simulink model "V1MatlabWs"  (R2019b)
settings: Solver=FixedStepAuto  StartTime=0.0  StopTime=20.0  FixedStep=0.1  MaxStep=0.1  MinStep=0.1  RelTol=1e-3  EnableMultiTasking=on
values from neighbouring files (symbols this model uses):
  c1 = c    (= 1)    [V1SetParam.m]    (also in V3VektorSetParam.m; V7Callback_2018_05_25_18_20_53_343.mat; V7SetParam.m; myData.mat)
  c2 = c    (= 1)    [V1SetParam.m]    (also in V3VektorSetParam.m; V7Callback_2018_05_25_18_20_53_343.mat; V7SetParam.m)
  c3 = c    (= 1)    [V1SetParam.m]    (also in V3VektorSetParam.m; V7Callback_2018_05_25_18_20_53_343.mat; V7SetParam.m)
  c4 = c    (= 1)    [V1SetParam.m]    (also in V3VektorSetParam.m; V7Callback_2018_05_25_18_20_53_343.mat; V7SetParam.m)
  m1 = m    (= 2)    [V1SetParam.m]    (also in V3VektorSetParam.m; V7Callback_2018_05_25_18_20_53_343.mat; V7SetParam.m; myData.mat)
  m2 = m    (= 2)    [V1SetParam.m]    (also in V3VektorSetParam.m; V7Callback_2018_05_25_18_20_53_343.mat; V7SetParam.m)
  m3 = m    (= 2)    [V1SetParam.m]    (also in V3VektorSetParam.m; V7Callback_2018_05_25_18_20_53_343.mat; V7SetParam.m)
  v1 = 0    [V7Callback_2018_05_25_18_20_53_343.mat]    (also in V7SetParam.m)
  v2 = 0    [V7Callback_2018_05_25_18_20_53_343.mat]    (also in V7SetParam.m)
  v3 = 0    [V7Callback_2018_05_25_18_20_53_343.mat]    (also in V7SetParam.m)
  x1 = -1    [V7Callback_2018_05_25_18_20_53_343.mat]    (also in V7SetParam.m)
  x2 = 0    [V7Callback_2018_05_25_18_20_53_343.mat]    (also in V7SetParam.m)
  x3 = 1    [V7Callback_2018_05_25_18_20_53_343.mat]    (also in V7SetParam.m)
settings Model: Creator=Reichl  LastModifiedBy=jakob
settings DataIOCC: SaveFormat=Array  SignalLoggingSaveFormat=ModelDataLogs  ReturnWorkspaceOutputs=off
settings OptimizationCC: ExpressionDepthLimit=2147483647  LifeSpan=inf
settings DebuggingCC: UnderspecifiedInitializationDetection=Classic  MergeDetectMultiDrivingBlocksExec=none  SolverPrmCheckMsg=warning  FcnCallInpInsideContextMsg=warning  AllowSymbolicDim=off  StateNameClashWarn=warning  SFUnexpectedBacktrackingDiag=warning  SFNoUnconditionalDefaultTransitionDiag=warning  SFExecutionAtInitializationDiag=none  ArithmeticOperatorsInVariantConditions=warning
settings HardwareCC: ProdBitPerPointer=32  ProdBitPerSizeT=32  ProdBitPerPtrDiffT=32  ProdLargestAtomicFloat=None  ProdIntDivRoundTo=Undefined  ProdEndianess=Unspecified  ProdWordSize=32  ProdHWDeviceType=32-bit Generic
settings ModelReferenceCC: PropagateSignalLabelsOutOfModel=off
settings SFSimCC: SimUseLocalCustomCode=off  CustomCodeUndefinedFunction=UseInterfaceOnly
settings RTWCC: RTWUseLocalCustomCode=off
settings CodeAppCC: StateflowObjectComments=on
settings GRTTargetCC: TargetLangStandard=C89/C90 (ANSI)  GeneratePreprocessorConditionals=Disable all  CombineOutputUpdateFcns=off  GRTInterface=on
settings ConfigComp: CovMetricSettings=dw  CovHtmlReporting=on  CovSaveCumulativeToWorkspaceVar=on  CovSaveSingleToWorkspaceVar=on  CovExternalEMLEnable=off  CovSFcnEnable=off

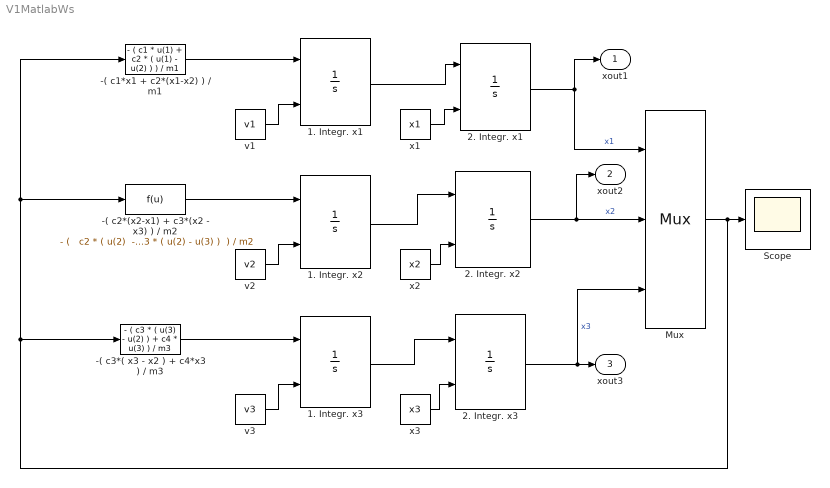
== system V1MatlabWs ==
  -( c1*x1 + c2*(x1-x2) ) / m1 : Fcn  Expr="- (   c1 * u(1)  +  c2 * ( u(1) - u(2) )  ) / m1"
  -( c2*(x2-x1) + c3*(x2 - x3) ) / m2 : Fcn  Expr="- (   c2 * ( u(2)  -u(1) )  +  c3 * ( u(2) - u(3) )  ) / m2"
  -( c3*( x3 - x2 ) + c4*x3 ) / m3 : Fcn  Expr="- (  c3 * ( u(3) - u(2) )  +  c4 * u(3)  ) / m3"
  1. Integr. x1 : Integrator  InitialConditionSource=external  InitialCondition=v1
  1. Integr. x2 : Integrator  InitialConditionSource=external  InitialCondition=v2
  1. Integr. x3 : Integrator  InitialConditionSource=external  InitialCondition=v3
  2. Integr. x1 : Integrator  InitialConditionSource=external  InitialCondition=x1
  2. Integr. x2 : Integrator  InitialConditionSource=external  InitialCondition=x2
  2. Integr. x3 : Integrator  InitialConditionSource=external  InitialCondition=x3
  Mux : Mux  Inputs=3
      settings: DisplayOption=signals
  Scope : Scope
  v1 : Constant  Value=v1
  v2 : Constant  Value=v2
  v3 : Constant  Value=v3
  x1 : Constant  Value=x1
  x2 : Constant  Value=x2
  x3 : Constant  Value=x3
  xout1 : Outport  VectorParamsAs1DForOutWhenUnconnected=off
  xout2 : Outport  Port=2  VectorParamsAs1DForOutWhenUnconnected=off
  xout3 : Outport  Port=3  VectorParamsAs1DForOutWhenUnconnected=off
  wires:
  1. Integr. x1/1 -> 2. Integr. x1/1
  1. Integr. x2/1 -> 2. Integr. x2/1
  1. Integr. x3/1 -> 2. Integr. x3/1
  Mux/1 -> Scope/1, -( c3*( x3 - x2 ) + c4*x3 ) / m3/1, -( c1*x1 + c2*(x1-x2) ) / m1/1, -( c2*(x2-x1) + c3*(x2 - x3) ) / m2/1
  2. Integr. x2/1 -> xout2/1, Mux/2  "x2"
  2. Integr. x1/1 -> xout1/1, Mux/1  "x1"
  2. Integr. x3/1 -> xout3/1, Mux/3  "x3"
  -( c1*x1 + c2*(x1-x2) ) / m1/1 -> 1. Integr. x1/1
  -( c2*(x2-x1) + c3*(x2 - x3) ) / m2/1 -> 1. Integr. x2/1
  -( c3*( x3 - x2 ) + c4*x3 ) / m3/1 -> 1. Integr. x3/1
  v1/1 -> 1. Integr. x1/2
  v2/1 -> 1. Integr. x2/2
  v3/1 -> 1. Integr. x3/2
  x1/1 -> 2. Integr. x1/2
  x3/1 -> 2. Integr. x3/2
  x2/1 -> 2. Integr. x2/2
